simulink model "final_model_birotor"  (Simulink 9.2)
settings: Solver=VariableStepAuto  StartTime=0.0  StopTime=250  RelTol=1e-3
undefined symbols (not defined in the file or in its folder): g, Iyy, kd, kp, l, m, Ts
libraries: simulink x2
settings Model: Creator=Mauri  LastModifiedBy=Mauri
settings Model: SuppressorTable=|
  | <?xml version="1.0" encoding="UTF-8" standalone="yes" ?>
  | <!DOCTYPE boost_serialization>
  | <boost_serialization signature="serialization::archive" version="15">
  | <DiagnosticSuppressor class_id="0" tracking_level="0" version="6">
  | 	<Table class_id="1" tracking_level="0" version="0">
  | 		<count>2</count>
  | 		<bucket_count>8</bucket_count>
  | 		<item_version>0</item_version>
  | 		<item class_id="2" tracking_level="0" version="0">
  | 			<first class_id="3" tracking_level="0" version="6">
  | 				<Source class_id="4" tracking_level="0" version="0">
  | 					<count>1</count>
  | 					<item_version>0</item_version>
  | 					<item>final_model_birotor/Ref_theta1/LimitedCounter</item>
  | 				</Source>
  | 			</first>
  | 			<second class_id="5" tracking_level="0" version="6">
  | 				<SuppressedData class_id="6" tracking_level="0" version="0">
  | 					<count>2</count>
  | 					<bucket_count>8</bucket_count>
  | 					<item_version>0</item_version>
  | 					<item class_id="7" tracking_level="0" version="0">
  | 						<first class_id="8" tracking_level="0" version="6">
  | 							<ID>SimulinkFixedPoint:util:Overflowoccurred</ID>
  | 							<Cause>
  | 								<Source>
  | 									<count>0</count>
  | 									<item_version>0</item_version>
  | 								</Source>
  | 							</Cause>
  | 						</first>
  | 						<second class_id="9" tracking_level="0" version="6">
  | 							<Comment></Comment>
  | 							<User></User>
  | 							<LastModified class_id="10" tracking_level="0" version="0">
  | 								<ptime_date class_id="11" tracking_level="0" version="0">
  | 									<date>20160608</date>
  | 								</ptime_date>
  | 								<ptime_time_duration class_id="12" tracking_level="0" version="0">
  | 									<is_special>0</is_special>
  | 									<time_duration_hours>15</time_duration_hours>
  | 									<time_duration_minutes>23</time_duration_minutes>
  | 									<time_duration_seconds>17</time_duration_seconds>
  | 									<time_duration_fractional_seconds>0</time_duration_fractional_seconds>
  | 								</ptime_time_duration>
  | 							</LastModified>
  | 							<SuppressionType>1</SuppressionType>
  | 						</second>
  | 					</item>
  | 					<item>
  | 						<first>
  | 							<ID>Simulink:DataType:WarningOverFlowDetected</ID>
  | 							<Cause>
  | 								<Source>
  | 									<count>0</count>
  | 									<item_version>0</item_version>
  | 								</Source>
  | 							</Cause>
  | 						</first>
  | 						<second>
  | 							<Comment></Comment>
  | 							<User></User>
  | 							<LastModified>
  | 								<ptime_date>
  | 									<date>20160608</date>
  | 								</ptime_date>
  | 								<ptime_time_duration>
  | 									<is_special>0</is_special>
  | 									<time_duration_hours>15</time_duration_hours>
  | 									<time_duration_minutes>23</time_duration_minutes>
  | 									<time_duration_seconds>17</time_duration_seconds>
  | 									<time_duration_fractional_seconds>0</time_duration_fractional_seconds>
  | 								</ptime_time_duration>
  | 							</LastModified>
  | 							<SuppressionType>1</SuppressionType>
  | 						</second>
  | 					</item>
  | 				</SuppressedData>
  | 			</second>
  | 		</item>
  | 		<item>
  | 			<first>
  | 				<Source>
  | 					<count>1</count>
  | 					<item_version>0</item_version>
  | 					<item>final_model_birotor/Ref_theta2/LimitedCounter</item>
  | 				</Source>
  | 			</first>
  | 			<second>
  | 				<SuppressedData>
  | 					<count>2</count>
  | 					<bucket_count>8</bucket_count>
  | 					<item_version>0</item_version>
  | 					<item>
  | 						<first>
  | 							<ID>SimulinkFixedPoint:util:Overflowoccurred</ID>
  | 							<Cause>
  | 								<Source>
  | 									<count>0</count>
  | 									<item_version>0</item_version>
  | 								</Source>
  | 							</Cause>
  | 						</first>
  | 						<second>
  | 							<Comment></Comment>
  | 							<User></User>
  | 							<LastModified>
  | 								<ptime_date>
  | 									<date>20160608</date>
  | 								</ptime_date>
  | 								<ptime_time_duration>
  | 									<is_special>0</is_special>
  | 									<time_duration_hours>15</time_duration_hours>
  | 									<time_duration_minutes>23</time_duration_minutes>
  | 									<time_duration_seconds>17</time_duration_seconds>
  | 									<time_duration_fractional_seconds>0</time_duration_fractional_seconds>
  | 								</ptime_time_duration>
  | 							</LastModified>
  | 							<SuppressionType>1</SuppressionType>
  | 						</second>
  | 					</item>
  | 					<item>
  | 						<first>
  | 							<ID>Simulink:DataType:WarningOverFlowDetected</ID>
  | 							<Cause>
  | 								<Source>
  | 									<count>0</count>
  | 									<item_version>0</item_version>
  | 								</Source>
  | 							</Cause>
  | 						</first>
  | 						<second>
  | 							<Comment></Comment>
  | 							<User></User>
  | 							<LastModified>
  | 								<ptime_date>
  | 									<date>20160608</date>
  | 								</ptime_date>
  | 								<ptime_time_duration>
  | 									<is_special>0</is_special>
  | 									<time_duration_hours>15</time_duration_hours>
  | 									<time_duration_minutes>23</time_duration_minutes>
  | 									<time_duration_seconds>17</time_duration_seconds>
  | 									<time_duration_fractional_seconds>0</time_duration_fractional_seconds>
  | 								</ptime_time_duration>
  | 							</LastModified>
  | 							<SuppressionType>1</SuppressionType>
  | 						</second>
  | 					</item>
  | 				</SuppressedData>
  | 			</second>
  | 		</item>
  | 	</Table>
  | </DiagnosticSuppressor>
  | </boost_serialization>
settings DataIOCC: LimitDataPoints=off  SaveFormat=Dataset  SignalLoggingSaveFormat=Dataset
settings OptimizationCC: LifeSpan=auto
settings DebuggingCC: UnderspecifiedInitializationDetection=Simplified  MergeDetectMultiDrivingBlocksExec=error  FcnCallInpInsideContextMsg=error  StateNameClashWarn=none  SFUnexpectedBacktrackingDiag=error  SFNoUnconditionalDefaultTransitionDiag=error  SFExecutionAtInitializationDiag=warning
settings HardwareCC: ProdBitPerPointer=64  ProdBitPerSizeT=64  ProdBitPerPtrDiffT=64  ProdLargestAtomicFloat=Float  ProdIntDivRoundTo=Zero  ProdEndianess=LittleEndian  ProdWordSize=64  ProdHWDeviceType=Intel->x86-64 (Windows64)
settings ModelReferenceCC: PropagateSignalLabelsOutOfModel=on
settings SFSimCC: SimUseLocalCustomCode=on
settings RTWCC: RTWUseLocalCustomCode=on
settings CodeAppCC: StateflowObjectComments=off
settings GRTTargetCC: TargetLangStandard=C99 (ISO)  GeneratePreprocessorConditionals=Use local settings  CombineOutputUpdateFcns=on  GRTInterface=off
settings ConfigComp: CovMetricSettings=dwe  CovHtmlReporting=off  CovSaveCumulativeToWorkspaceVar=off  CovSaveSingleToWorkspaceVar=off  CovExternalEMLEnable=on

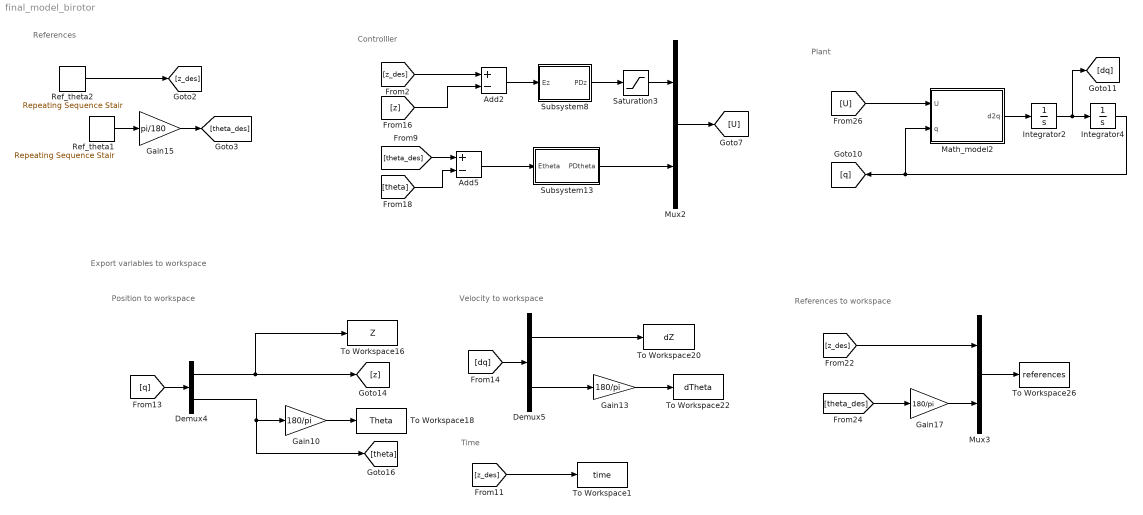
== system final_model_birotor ==
  note: Time
  note: Export variables to workspace
  note: Plant
  note: Controlller
  note: References
  note: Velocity to workspace
  note: Position to workspace
  note: References to workspace
  Add2 : Sum  Inputs=+-
  Add5 : Sum  Inputs=+-
  Demux4 : Demux  Outputs=2
  Demux5 : Demux  Outputs=2
  Gain10 : Gain  Gain=180/pi
  Gain13 : Gain  Gain=180/pi
  Gain15 : Gain  Gain=pi/180
  Gain17 : Gain  Gain=180/pi
  Integrator2 : Integrator
  Integrator4 : Integrator
  Math_model2 : MATLAB Function  TreatAsAtomicUnit=on
  Mux2 : Mux  Inputs=2
  Mux3 : Mux  Inputs=2
  Ref_theta1 : simulink/Sources/Repeating Sequence Stair  OutValues=[10 10 1 1 1 5 5 2 2 10 10 2 2].'  tsamp=10  OutMin=[]  OutMax=[]  OutDataTypeStr=double  OutputDataTypeScalingMode=double  OutDataType=fixdt(0,8)  ConRadixGroup=Best Precision: Vector-wise  OutScaling=2^-12
  Ref_theta2 : simulink/Sources/Repeating Sequence Stair  OutValues=[0.1 0.1 0.15 0.25 0.25 0.1 0.1 0.25 0.2 0.2 0.1 0.15].'  tsamp=10  OutMin=[]  OutMax=[]  OutDataTypeStr=double  OutputDataTypeScalingMode=double  OutDataType=fixdt(0,8)  ConRadixGroup=Best Precision: Vector-wise  OutScaling=2^-12
  Saturation3 : Saturate  UpperLimit=1000  LowerLimit=0
  Subsystem13 : Subsystem
  Subsystem8 : Subsystem
  To Workspace1 : ToWorkspace  VariableName=time  SaveFormat=Timeseries  SampleTime=Ts
  To Workspace16 : ToWorkspace  VariableName=Z  SampleTime=Ts
  To Workspace18 : ToWorkspace  VariableName=Theta  SampleTime=Ts
  To Workspace20 : ToWorkspace  VariableName=dZ  SampleTime=Ts
  To Workspace22 : ToWorkspace  VariableName=dTheta  SampleTime=Ts
  To Workspace26 : ToWorkspace  VariableName=references  SampleTime=Ts
  wires:
  Ref_theta1/1 -> Gain15/1
  Gain15/1 -> [theta_des]
  [z_des] -> Add2/1
  Subsystem8/1(PDz) -> Saturation3/1
  [z] -> Add2/2
  Add2/1 -> Subsystem8/1(Ez)
  Saturation3/1 -> Mux2/1
  [theta_des] -> Add5/1
  Subsystem13/1(PDtheta) -> Mux2/2
  Add5/1 -> Subsystem13/1(Etheta)
  [theta] -> Add5/2
  Mux2/1 -> [U]
  [U] -> Math_model2/1(U)
  [q] -> Demux4/1
  Demux5/2 -> Gain13/1
  Gain17/1 -> Mux3/2
  Mux3/1 -> To Workspace26/1
  Demux4/1 -> [z], To Workspace16/1
  [z_des] -> Mux3/1
  Demux4/2 -> [theta], Gain10/1
  Gain13/1 -> To Workspace22/1
  [dq] -> Demux5/1
  Gain10/1 -> To Workspace18/1
  [theta_des] -> Gain17/1
  Demux5/1 -> To Workspace20/1
  Integrator2/1 -> Integrator4/1, [dq]
  Math_model2/1(d2q) -> Integrator2/1
  [z_des] -> To Workspace1/1
  Integrator4/1 -> Math_model2/2(q), [q]
  Ref_theta2/1 -> [z_des]

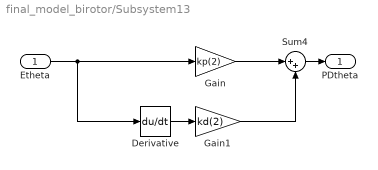
== system final_model_birotor/Subsystem13 ==
  Etheta : Inport
  Derivative : Derivative  CoefficientInTFapproximation=1
  Gain : Gain  Gain=kp(2)
  Gain1 : Gain  Gain=kd(2)
  Sum4 : Sum  Inputs=|++
  PDtheta : Outport
  wires:
  Gain1/1 -> Sum4/2
  Sum4/1 -> PDtheta/1
  Etheta/1 -> Gain/1, Derivative/1
  Derivative/1 -> Gain1/1
  Gain/1 -> Sum4/1

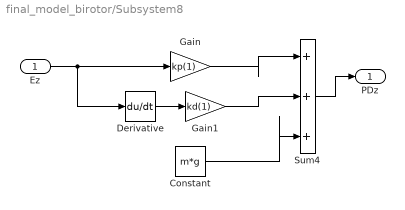
== system final_model_birotor/Subsystem8 ==
  Ez : Inport
  Constant : Constant  Value=m*g
  Derivative : Derivative  CoefficientInTFapproximation=1
  Gain : Gain  Gain=kp(1)
  Gain1 : Gain  Gain=kd(1)
  Sum4 : Sum  Inputs=|+++|
  PDz : Outport
  wires:
  Gain1/1 -> Sum4/2
  Derivative/1 -> Gain1/1
  Sum4/1 -> PDz/1
  Ez/1 -> Gain/1, Derivative/1
  Gain/1 -> Sum4/1
  Constant/1 -> Sum4/3

== matlab function Math_model2 ==
  data: U input double size=2,1; q input double; m parameter double; g parameter double; Iyy parameter double; d2q output double size=2,1; l parameter double
function d2q = model(U,q, m, g, Iyy, l)
%% Drone's Math model considering the Equations of Newton-Euler.
% Constants:
%   
%   m: Drone's mass
%   g: Gravity force
%   Iyy: Drone's moment of inertia about axis y
%   b: Trust constant.
%   d: Drug coefficient.
% Inputs: 
% Control signals
%       U1: z attitude control.
%       U2: pitch pd control.
% Outputs:
%       q(1): z earth frame position.
%       q(2): pitch angle.

% Euler angles.
theta = q(2);     % Pitch angle.

% Define the forces and torques about body frame.
d2z =-g+ (1/m)*cos(theta)*U(1);          % acceleration Z earth frame.
d2theta = (l/Iyy)*U(2);            % angular acceleration about y axis.
d2q = [d2z;d2theta];
